simulink model "exaulasimulacao"  (R2022a)
settings: Solver=VariableStepAuto  StartTime=0.0  StopTime=10  RelTol=1e-3
settings Model: Creator=a2150336  LastModifiedBy=a2150336

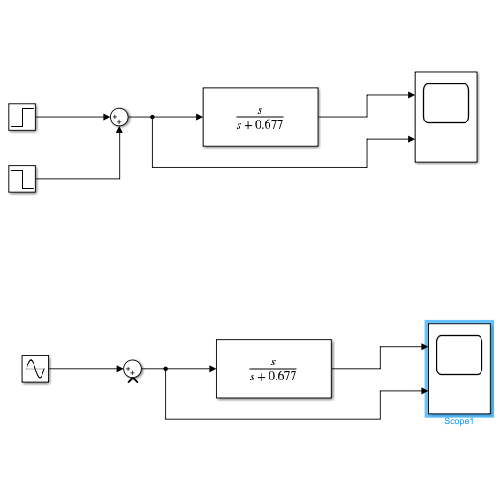
[thumbnail: Simulink's stored preview of the top-level diagram]
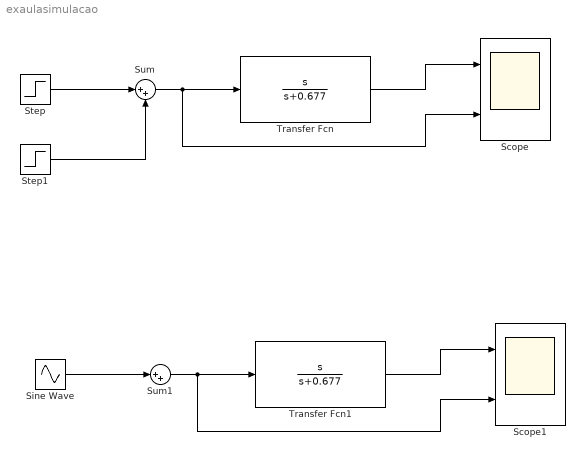
== system exaulasimulacao ==
  Scope : Scope  NumInputPorts=2
  Scope1 : Scope  NumInputPorts=2
  Sine Wave : Sin  SampleTime=0
  Step : Step  After=0.01  SampleTime=0
  Step1 : Step  Time=2  After=-0.02  SampleTime=0
  Sum : Sum  Inputs=|++
  Sum1 : Sum  Inputs=|++
  Transfer Fcn : TransferFcn  Numerator=[1 0]  Denominator=[1 0.677]
  Transfer Fcn1 : TransferFcn  Numerator=[1 0]  Denominator=[1 0.677]
  wires:
  Transfer Fcn/1 -> Scope/1
  Sum/1 -> Scope/2, Transfer Fcn/1
  Step/1 -> Sum/1
  Step1/1 -> Sum/2
  Sum1/1 -> Scope1/2, Transfer Fcn1/1
  Transfer Fcn1/1 -> Scope1/1
  Sine Wave/1 -> Sum1/1
